simulink model "tes"  (R2023b)
settings: Solver=VariableStepAuto  StartTime=0.0  StopTime=10  RelTol=1e-3
values from neighbouring files (symbols this model uses):
  A = [0, 0, 1, 0 ... (first row only)    [Continuous_state_space_model.m]
  B = [0; 0; 1/mc; 1/ (L*mc) ]    [Continuous_state_space_model.m]
  K = acker(A,B,des_pole)    [Continuous_state_space_model.m]
settings Model: Creator=Gabriel  LastModifiedBy=Jonathan

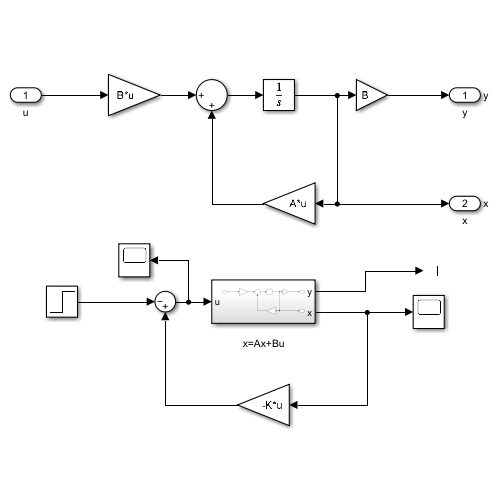
[thumbnail: Simulink's stored preview of the top-level diagram]
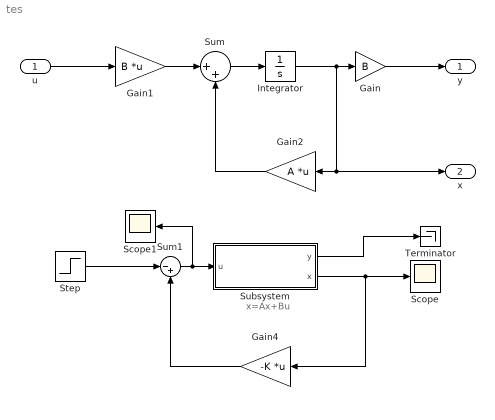
== system tes ==
  note: x=Ax+Bu
  u : Inport
  Gain : Gain  Gain=B
  Gain1 : Gain  Gain=B  Multiplication=Matrix(K*u)
  Gain2 : Gain  Gain=A  Multiplication=Matrix(K*u)
  Gain4 : Gain  Gain=-K  Multiplication=Matrix(K*u)
  Integrator : Integrator
  Scope : Scope
  Scope1 : Scope
  Step : Step  Time=0  SampleTime=0
  Subsystem : Subsystem
  Sum : Sum  Inputs=|++
  Sum1 : Sum  Inputs=|-+
  Terminator : Terminator
  y : Outport  SignalName=y
  x : Outport  Port=2  SignalName=x
  wires:
  u/1 -> Gain1/1
  Gain1/1 -> Sum/1
  Sum/1 -> Integrator/1
  Integrator/1 -> x/1, Gain2/1, Gain/1
  Gain/1 -> y/1
  Subsystem/1(y) -> Terminator/1
  Gain2/1 -> Sum/2
  Subsystem/2(x) -> Gain4/1, Scope/1
  Gain4/1 -> Sum1/2
  Step/1 -> Sum1/1
  Sum1/1 -> Scope1/1, Subsystem/1(u)

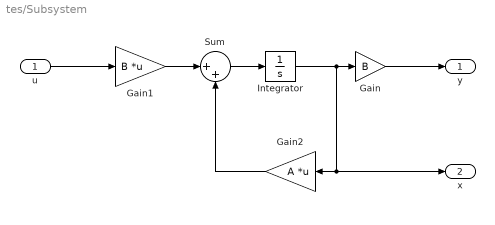
== system tes/Subsystem ==
  u : Inport
  Gain : Gain  Gain=B
  Gain1 : Gain  Gain=B  Multiplication=Matrix(K*u)
  Gain2 : Gain  Gain=A  Multiplication=Matrix(K*u)
  Integrator : Integrator
  Sum : Sum  Inputs=|++
  y : Outport
  x : Outport  Port=2
  wires:
  Gain2/1 -> Sum/2
  Gain/1 -> y/1
  Integrator/1 -> x/1, Gain2/1, Gain/1
  u/1 -> Gain1/1
  Sum/1 -> Integrator/1
  Gain1/1 -> Sum/1
